simulink model "model_chap8"  (R2018a)
settings: Solver=VariableStepAuto  StartTime=0.0  StopTime=10.0  RelTol=1e-3
values from neighbouring files (symbols this model uses):
  a = 20.2    [Chapter6.m]    (also in Chapter6_bis.m; Chapter8.m)
  A_R = [A_longitude_lo(1,1:5) ; A_longitude_lo(2,1:5) ; A_longitude_lo(3,1:5) ; A_longitude_lo(4,1:5) ; A_longitude_lo(5,1:5)]    [Chapter8.m]
  B_R = [A_longitude_lo(1,  7) ; A_longitude_lo(2,  7) ; A_longitude_lo(3,  7) ; A_longitude_lo(4,  7) ; A_longitude_lo(5,  7)]    [Chapter8.m]
  C_R = [C_longitude_lo(1,1:5) ; C_longitude_lo(2,1:5) ; C_longitude_lo(3,1:5) ; C_longitude_lo(4,1:5) ; C_longitude_lo(5,1:5)]    [Chapter8.m]
  D_R = zeros(5,1)    [Chapter8.m]
settings Model: Creator=Alex  LastModifiedBy=Alex

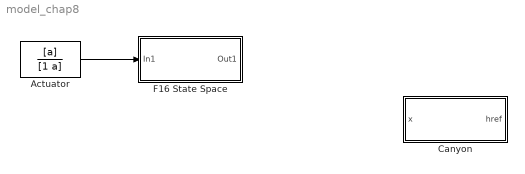
== system model_chap8 ==
  Actuator : TransferFcn  Numerator=[a]  Denominator=[1 a]
  Canyon : Subsystem
  F16 State Space : Subsystem
  wires:
  Actuator/1 -> F16 State Space/1(In1)

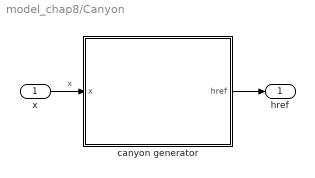
== system model_chap8/Canyon ==
  x : Inport
  canyon generator : Subsystem
      mask Display: image(imread('refalt.jpg'))
  href : Outport
  wires:
  x/1 -> canyon generator/1(x)  "x"
  canyon generator/1(href) -> href/1

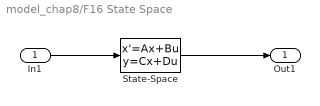
== system model_chap8/F16 State Space ==
  In1 : Inport
  State-Space : StateSpace  A=A_R  B=B_R  C=C_R  D=D_R  InitialCondition=0
  Out1 : Outport
  wires:
  State-Space/1 -> Out1/1
  In1/1 -> State-Space/1

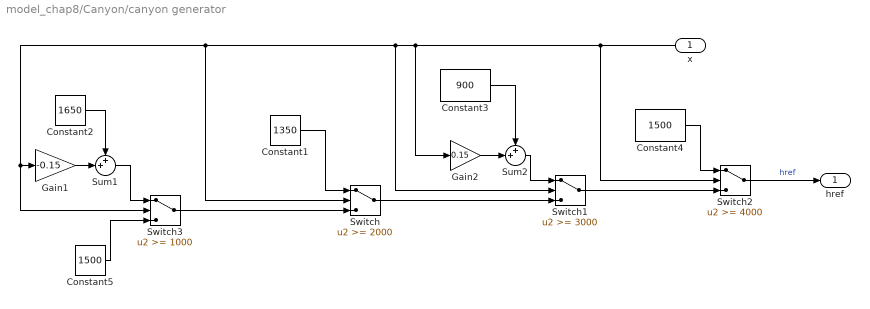
== system model_chap8/Canyon/canyon generator ==
  x : Inport
  Constant1 : Constant  Value=1350
  Constant2 : Constant  Value=1650
  Constant3 : Constant  Value=900
  Constant4 : Constant  Value=1500
  Constant5 : Constant  Value=1500
  Gain1 : Gain  Gain=-0.15
  Gain2 : Gain  Gain=0.15
  Sum1 : Sum  Inputs=++|
  Sum2 : Sum  Inputs=++|
  Switch : Switch  Threshold=2000  ZeroCross=off
  Switch1 : Switch  Threshold=3000  ZeroCross=off
  Switch2 : Switch  Threshold=4000  ZeroCross=off
  Switch3 : Switch  Threshold=1000  ZeroCross=off
  href : Outport
  wires:
  Constant1/1 -> Switch/1
  x/1 -> Switch2/2, Gain2/1, Switch1/2, Switch/2, Gain1/1, Switch3/2
  Switch/1 -> Switch1/3
  Gain2/1 -> Sum2/2
  Constant3/1 -> Sum2/1
  Sum2/1 -> Switch1/1
  Switch1/1 -> Switch2/3
  Constant4/1 -> Switch2/1
  Switch2/1 -> href/1  "href"
  Switch3/1 -> Switch/3
  Constant5/1 -> Switch3/3
  Sum1/1 -> Switch3/1
  Gain1/1 -> Sum1/2
  Constant2/1 -> Sum1/1
